simulink model "CL_pi_testExecutionMutants"  (R2017b)
settings: Solver=ode3  StartTime=0.0  StopTime=inf  FixedStep=ts  RelTol=0.01  EnableMultiTasking=on
InitFcn:
  | ts=0.0005
  | %ts=100e-6;
StartFcn:
  | close all
StopFcn:
  | % Speed Torque Characterstic
  | 
  | 
  | %figure('Units','pixels', ...
  | %'Color',[1 1 1], ...
  | %'Name','Speed Torque Characterstic',...
  | %'NumberTitle','off',...
  | %'Position',[400 50 470 300], ...
  | %'ToolBar','none');
  | 
  | 
  | 
  | %plot(N_pi,Te_pi)
  | %title('Speed Torque Characterstic')
  | %xlabel('Speed [ RPM ]')
  | %ylabel('Electromagnetic Te_pi [ Nm ] ')
  | %grid on
  | %clear p4 p7 param5 param6 param8 parametres visible voltage
  | 
  | 
  | %clc
values from neighbouring files (symbols this model uses):
  TestOrder = [i]    [ExecuteTestSuite.m]    (also in mutants.m)
undefined symbols (not defined in the file or in its folder): emergency_button2, emergency_buttons, tc_simul, tc_size, temperature, trans1, trans2, trans3, trans4
libraries: simulink x48, powerlib_extras x12
(part 6 of 6)

== system CL_pi_testExecutionMutants/mutant3/VSI/SPWM/Carier Wave Signal ==
  Carier Wave : simulink/Sources/Repeating Sequence  rep_seq_t=[0 0.25 0.5 0.75 1]./fc  rep_seq_y=[0 1 0 -1 0].*A
  "Carier Wave " : Outport
  wires:
  Carier Wave/1 -> "Carier Wave "/1  "0 delay"

== system CL_pi_testExecutionMutants/mutant4/VSI/SPWM/Carier Wave Signal ==
  Carier Wave : simulink/Sources/Repeating Sequence  rep_seq_t=[0 0.25 0.5 0.75 1]./fc  rep_seq_y=[0 1 0 -1 0].*A
  "Carier Wave " : Outport
  wires:
  Carier Wave/1 -> "Carier Wave "/1  "0 delay"

== system CL_pi_testExecutionMutants/mutant5/VSI/SPWM/Carier Wave Signal ==
  Carier Wave : simulink/Sources/Repeating Sequence  rep_seq_t=[0 0.25 0.5 0.75 1]./fc  rep_seq_y=[0 1 0 -1 0].*A
  "Carier Wave " : Outport
  wires:
  Carier Wave/1 -> "Carier Wave "/1  "0 delay"

== system CL_pi_testExecutionMutants/mutant6/VSI/SPWM/Carier Wave Signal ==
  Carier Wave : simulink/Sources/Repeating Sequence  rep_seq_t=[0 0.25 0.5 0.75 1]./fc  rep_seq_y=[0 1 0 -1 0].*A
  "Carier Wave " : Outport
  wires:
  Carier Wave/1 -> "Carier Wave "/1  "0 delay"

== system CL_pi_testExecutionMutants/mutant7/VSI/SPWM/Carier Wave Signal ==
  Carier Wave : simulink/Sources/Repeating Sequence  rep_seq_t=[0 0.25 0.5 0.75 1]./fc  rep_seq_y=[0 1 0 -1 0].*A
  "Carier Wave " : Outport
  wires:
  Carier Wave/1 -> "Carier Wave "/1  "0 delay"

== system CL_pi_testExecutionMutants/mutant8/VSI/SPWM/Carier Wave Signal ==
  Carier Wave : simulink/Sources/Repeating Sequence  rep_seq_t=[0 0.25 0.5 0.75 1]./fc  rep_seq_y=[0 1 0 -1 0].*A
  "Carier Wave " : Outport
  wires:
  Carier Wave/1 -> "Carier Wave "/1  "0 delay"

== system CL_pi_testExecutionMutants/mutant9/VSI/SPWM/Carier Wave Signal ==
  Carier Wave : simulink/Sources/Repeating Sequence  rep_seq_t=[0 0.25 0.5 0.75 1]./fc  rep_seq_y=[0 1 0 -1 0].*A
  "Carier Wave " : Outport
  wires:
  Carier Wave/1 -> "Carier Wave "/1  "0 delay"

== matlab function CL_pi_testExecutionMutants/TestExecutor/MATLAB Function ==
  data: tc_simul input; port_1 output; test_case input; state input; port_2 output; port_3 output; port_4 output
function [port_1,port_2,port_3,port_4] = fcn(tc_simul, test_case, state)
%#codegen
    port_1 = tc_simul(test_case, 4*(state-1)+1);
    port_2 = tc_simul(test_case, 4*(state-1)+2);
    port_3 = tc_simul(test_case, 4*(state-1)+3);
    port_4 = tc_simul(test_case, 4*(state-1)+4);


end

== matlab function CL_pi_testExecutionMutants/TestExecutor/MATLAB Function1 ==
  data: test_order input; tc_size input; trans1 input; trans2 input; trans3 input; trans4 input; v_engine input; temp input; test_order_id input; state_id input; test_case output; state output; test_order_id1 output; state_id1 output; simulation_stop output
function [test_case, state, test_order_id1, state_id1,simulation_stop] = fcn(test_order, tc_size, trans1,trans2, trans3, trans4, v_engine, temp,test_order_id,state_id)
%#codegen
    num_signals = 4;
    test_case = test_order(test_order_id);
    test_order_id1 = test_order_id;
    state = state_id;
    state_id1 = state;
    simulation_stop = false;
    
    if v_engine > trans1(test_case,state_id) && v_engine < trans2(test_case,state_id)
       if state_id<tc_size(test_case)/num_signals
          state = state_id+1;
          state_id1 = state;
       else
           if test_order_id1 < size(test_order,1)
               state = 1;
               state_id1 = state;
               test_order_id1 = test_order_id + 1;
           else
               simulation_stop = true;
               
           end
       end
    end

end
